simulink library "simCryogenics_lib"  (R2016a)
settings: Solver=VariableStepAuto  StartTime=0.0  StopTime=10.0  RelTol=1e-3
undefined symbols (not defined in the file or in its folder): gcbh, simscape
(part 1 of 4)
settings Model: Creator=FB229602  LastModifiedBy=FB229602
settings GRTTargetCC: GeneratePreprocessorConditionals=Use local settings

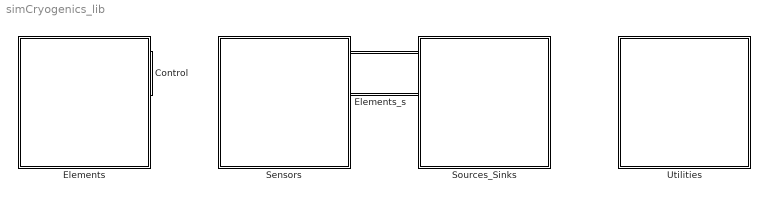
== system simCryogenics_lib ==
  Control : Subsystem  Tag=simscape_sublibrary
      mask Display: disp(get_param(gcb,'Name'))
  Elements : Subsystem  Tag=simscape_sublibrary
      mask Display: image(nesl_icon(gcb, 'simCryogenics.Elements.lib', '.m', '.png', 0, 2))
  Elements_s : Subsystem  Tag=simscape_sublibrary
      mask Display: disp(get_param(gcb,'Name'))
  Sensors : Subsystem  Tag=simscape_sublibrary
      mask Display: image(nesl_icon(gcb, 'simCryogenics.Sensors.lib', '.m', '.png', 0, 2))
  Sources_Sinks : Subsystem  Tag=simscape_sublibrary
      mask Display: image(nesl_icon(gcb, 'simCryogenics.Sources_Sinks.lib', '.m', '.png', 0, 2))
  Utilities : Subsystem  Tag=simscape_sublibrary
      mask Display: image(nesl_icon(gcb, 'simCryogenics.Utilities.lib', '.m', '.png', 0, 2))

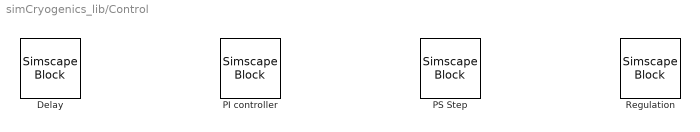
== system simCryogenics_lib/Control ==
  Delay : SimscapeBlock  DialogController=NetworkEngine.DynNeDlgSource  LoadFcn=simscape.compiler.sli.internal.callback('LoadFcn',gcbh);  SourceFile=simCryogenics.Control.Delay  mask(Delay){ComponentPath=simCryogenics.Control.Delay, ComponentVariants=simCryogenics.Control.Delay, ComponentVariantNames=Delay, ClassName=Delay, SchemaVersion=1, InputHistory=0.0, InputHistory_unit=1, InputHistory_conf=compiletime, DelayTime=1.0, DelayTime_unit=s, DelayTime_conf=compiletime}
      mask prompts: InputHistory "Input history"; DelayTime "Delay time"
      mask help: This block returns the input signal delayed by the specified time.
      mask init:
      | simscape.compiler.sli.internal.preinitmask(gcb);
      settings: CopyFcn=simscape.compiler.sli.internal.callback('CopyFcn',gcbh);  DeleteFcn=simscape.compiler.sli.internal.callback('DeleteFcn',gcbh);  ModelCloseFcn=simscape.compiler.sli.internal.callback('ModelCloseFcn',gcbh);  PreSaveFcn=simscape.compiler.sli.internal.callback('PreSaveFcn',gcbh);  PostSaveFcn=simscape.compiler.sli.internal.callback('PostSaveFcn',gcbh);  PreCopyFcn=simscape.compiler.sli.internal.callback('PreCopyFcn',gcbh);  PreDeleteFcn=simscape.compiler.sli.internal.callback('PreDeleteFcn',gcbh);
      mask Help: web(nesl_help(gcbh))
      mask TypeOptions InputHistory_conf: compiletime | runtime
      mask TypeOptions DelayTime_conf: compiletime | runtime
      mask Display:
      | disp('Simscape\n\n\n')
      | disp('\n\n\nDelay');
      | color('red');
      | port_label('RConn', 1,'Y');
      | port_label('LConn', 1,'U');
  PI controller : SimscapeBlock  DialogController=NetworkEngine.DynNeDlgSource  LoadFcn=simscape.compiler.sli.internal.callback('LoadFcn',gcbh);  SourceFile=simCryogenics.Control.PI  mask(PI controller){ComponentPath=simCryogenics.Control.PI, ComponentVariants=simCryogenics.Control.PI, ComponentVariantNames=PI, ClassName=PI, SchemaVersion=1, ctrl_type=0, ctrl_type_unit=1, ctrl_type_conf=compiletime, p_gain=1, p_gain_unit=1, p_gain_conf=compiletime, i_gain=1, i_gain_unit=1/s, i_gain_conf=compiletime, offset=1, offset_unit=1, offset_conf=compiletime, sat_min=- 1e9, sat_min_unit=1, sat_min_conf=compiletime, sat_max=+ 1e9, sat_max_unit=1, sat_max_conf=compiletime, c_PC_specify=off, c_PC_priority=None, c_PC=0, c_PC_unit=1, err_specify=off, err_priority=None, err=0, err_unit=1, errDer_specify=off, errDer_priority=None, errDer=0, errDer_unit=1}
      mask prompts: ctrl_type "Controller type"; p_gain "Proportional gain"; i_gain "Integral gain"; offset "PC offset"; sat_min "PC saturation minimum"; sat_max "PC saturation maximum"; c_PC_specify "c_PC"; c_PC_priority "c_PC"; err_specify "err"; err_priority "err"; errDer_specify "errDer"; errDer_priority "errDer"
      mask help: This regulation bloc implements a simple P controller by multiplying the error relative to the reference and adding the result with a specified offset. Input p_v (measure) should be connected to a physical signal from a sensor. Input f_c (final command) is the constant command to be applied after switch time. Output p_c (command) is the resulting command. Parameter st (switch time) is the time at which you want to switch to a constant command when the simulation time exceeds st, the regulation will be turned off and the specified constant command will be applied.
      mask init:
      | simscape.compiler.sli.internal.preinitmask(gcb);
      settings: CopyFcn=simscape.compiler.sli.internal.callback('CopyFcn',gcbh);  DeleteFcn=simscape.compiler.sli.internal.callback('DeleteFcn',gcbh);  ModelCloseFcn=simscape.compiler.sli.internal.callback('ModelCloseFcn',gcbh);  PreSaveFcn=simscape.compiler.sli.internal.callback('PreSaveFcn',gcbh);  PostSaveFcn=simscape.compiler.sli.internal.callback('PostSaveFcn',gcbh);  PreCopyFcn=simscape.compiler.sli.internal.callback('PreCopyFcn',gcbh);  PreDeleteFcn=simscape.compiler.sli.internal.callback('PreDeleteFcn',gcbh);
      mask Help: web(nesl_help(gcbh))
      mask TypeOptions ctrl_type_conf: compiletime | runtime
      mask TypeOptions p_gain_conf: compiletime | runtime
      mask TypeOptions i_gain_conf: compiletime | runtime
      mask TypeOptions offset_conf: compiletime | runtime
      mask TypeOptions sat_min_conf: compiletime
      mask TypeOptions sat_max_conf: compiletime
      mask TypeOptions c_PC_priority: None | Low | High
      mask TypeOptions err_priority: None | Low | High
      mask TypeOptions errDer_priority: None | Low | High
      mask Display:
      | disp('Simscape\n\n\n')
      | disp('\n\n\nPI');
      | color('red');
      | port_label('RConn', 1,'PC');
      | port_label('LConn', 3,'SP');
      | port_label('LConn', 2,'Tr');
      | port_label('LConn', 1,'PV');
  PS Step : SimscapeBlock  DialogController=NetworkEngine.DynNeDlgSource  LoadFcn=simscape.compiler.sli.internal.callback('LoadFcn',gcbh);  SourceFile=simCryogenics.Control.step  mask(PS Step){ComponentPath=simCryogenics.Control.step, ComponentVariants=simCryogenics.Control.step, ComponentVariantNames=step, ClassName=step, SchemaVersion=1, init_val=0, init_val_unit=1, init_val_conf=compiletime, final_val=1, final_val_unit=1, final_val_conf=compiletime, step_time=1, step_time_unit=1, step_time_conf=compiletime}
      mask prompts: init_val "Initial output value"; final_val "Final output value"; step_time "Step time"
      mask help: This component outputs a physical signal step from init_val to final_val at specified time step_time.
      mask init:
      | simscape.compiler.sli.internal.preinitmask(gcb);
      settings: CopyFcn=simscape.compiler.sli.internal.callback('CopyFcn',gcbh);  DeleteFcn=simscape.compiler.sli.internal.callback('DeleteFcn',gcbh);  ModelCloseFcn=simscape.compiler.sli.internal.callback('ModelCloseFcn',gcbh);  PreSaveFcn=simscape.compiler.sli.internal.callback('PreSaveFcn',gcbh);  PostSaveFcn=simscape.compiler.sli.internal.callback('PostSaveFcn',gcbh);  PreCopyFcn=simscape.compiler.sli.internal.callback('PreCopyFcn',gcbh);  PreDeleteFcn=simscape.compiler.sli.internal.callback('PreDeleteFcn',gcbh);
      mask Help: web(nesl_help(gcbh))
      mask TypeOptions init_val_conf: compiletime | runtime
      mask TypeOptions final_val_conf: compiletime | runtime
      mask TypeOptions step_time_conf: compiletime | runtime
      mask Display:
      | disp('Simscape\n\n\n')
      | disp('\n\n\nstep');
      | color('red');
      | port_label('RConn', 1,'out');
  Regulation : SimscapeBlock  DialogController=NetworkEngine.DynNeDlgSource  LoadFcn=simscape.compiler.sli.internal.callback('LoadFcn',gcbh);  SourceFile=simCryogenics.Control.regul  mask(Regulation){ComponentPath=simCryogenics.Control.regul, ComponentVariants=simCryogenics.Control.regul, ComponentVariantNames=regul, ClassName=regul, SchemaVersion=1, ctrl_type=0, ctrl_type_unit=1, ctrl_type_conf=compiletime, reference=1, reference_unit=1, reference_conf=compiletime, p_gain=1, p_gain_unit=1, p_gain_conf=compiletime, i_gain=1, i_gain_unit=1/s, i_gain_conf=compiletime, offset=1, offset_unit=1, offset_conf=compiletime, sat_min=- 1e9, sat_min_unit=1, sat_min_conf=compiletime, sat_max=+ 1e9, sat_max_unit=1, sat_max_conf=compiletime, switch_time=1e9, switch_time_unit=1, switch_time_conf=compiletime, c_command_specify=off, c_command_priority=None, c_command=0, c_command_unit=1, err_specify=off, err_priority=None, err=0, err_unit=1, errDer_specify=off, errDer_priority=None, errDer=0, errDer_unit=1}
      mask prompts: ctrl_type "Controller type"; reference "Reference to follow"; p_gain "Proportional gain"; i_gain "Integral gain"; offset "Command offset"; sat_min "Command saturation minimum"; sat_max "Command saturation maximum"; switch_time "Time after which the regulation will be turned off"; c_command_specify "c_command"; c_command_priority "c_command"; err_specify "err"; err_priority "err"; errDer_specify "errDer"; errDer_priority "errDer"
      mask help: This regulation bloc implements a simple P controller by multiplying the error relative to the reference and adding the result with a specified offset. Input p_v (measure) should be connected to a physical signal from a sensor. Input f_c (final command) is the constant command to be applied after switch time. Output p_c (command) is the resulting command. Parameter st (switch time) is the time at which you want to switch to a constant command when the simulation time exceeds st, the regulation will be turned off and the specified constant command will be applied.
      mask init:
      | simscape.compiler.sli.internal.preinitmask(gcb);
      settings: CopyFcn=simscape.compiler.sli.internal.callback('CopyFcn',gcbh);  DeleteFcn=simscape.compiler.sli.internal.callback('DeleteFcn',gcbh);  ModelCloseFcn=simscape.compiler.sli.internal.callback('ModelCloseFcn',gcbh);  PreSaveFcn=simscape.compiler.sli.internal.callback('PreSaveFcn',gcbh);  PostSaveFcn=simscape.compiler.sli.internal.callback('PostSaveFcn',gcbh);  PreCopyFcn=simscape.compiler.sli.internal.callback('PreCopyFcn',gcbh);  PreDeleteFcn=simscape.compiler.sli.internal.callback('PreDeleteFcn',gcbh);
      mask Help: web(nesl_help(gcbh))
      mask TypeOptions ctrl_type_conf: compiletime | runtime
      mask TypeOptions reference_conf: compiletime | runtime
      mask TypeOptions p_gain_conf: compiletime | runtime
      mask TypeOptions i_gain_conf: compiletime | runtime
      mask TypeOptions offset_conf: compiletime | runtime
      mask TypeOptions sat_min_conf: compiletime
      mask TypeOptions sat_max_conf: compiletime
      mask TypeOptions switch_time_conf: compiletime
      mask TypeOptions c_command_priority: None | Low | High
      mask TypeOptions err_priority: None | Low | High
      mask TypeOptions errDer_priority: None | Low | High
      mask Display:
      | disp('Simscape\n\n\n')
      | disp('\n\n\nregul');
      | color('red');
      | port_label('RConn', 1,'PC');
      | port_label('LConn', 2,'f_c');
      | port_label('LConn', 1,'PV');
